simulink model "my_queue_system"  (R2023a)
settings: Solver=VariableStepAuto  StartTime=0.0  StopTime=1000  RelTol=1e-3
values from neighbouring files (symbols this model uses):
  m = m + 1    (= 2)    [TMO5liubimov.m]    (also in laba2.m = 14; laba3.m = 200; test.m = 5)
  n = 31    [laba2.m]    (also in test.m = 7)
settings Model: PacingRate=14  Creator=PC  LastModifiedBy=PC

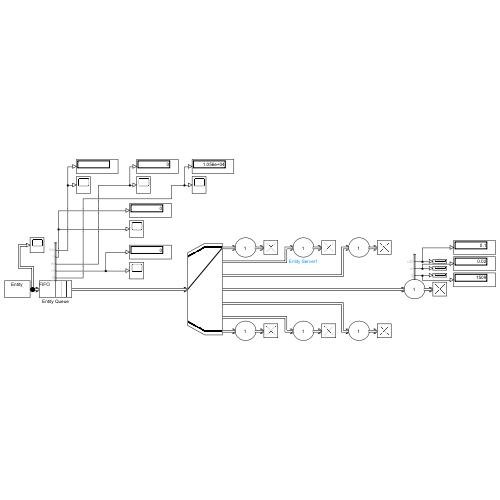
[thumbnail: Simulink's stored preview of the top-level diagram]
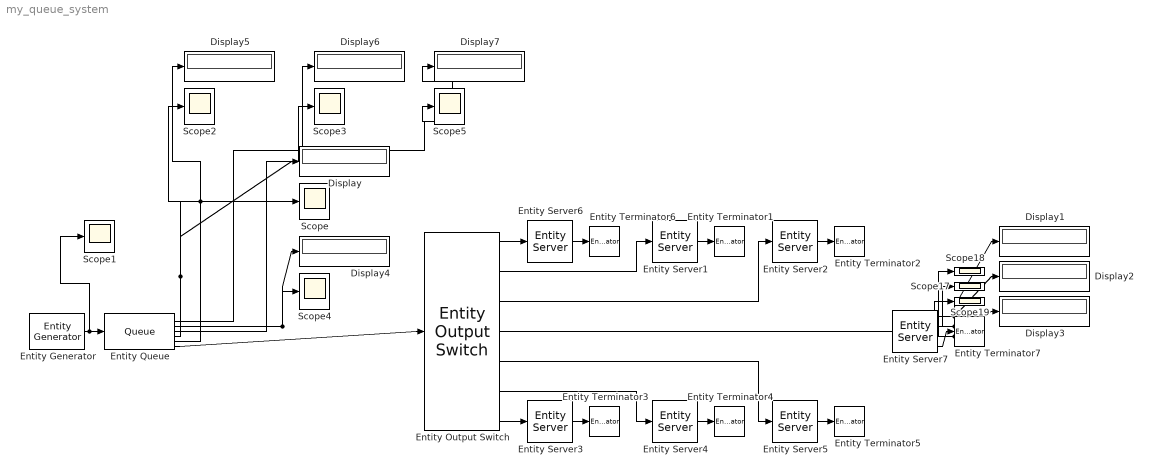
== system my_queue_system ==
  Display{,1..7} (8 alike) : Display
  Entity Output Switch : EntityOutputSwitch  InputPortMessageModes=m  OutputPortMessageModes=m,m,m,m,m,m,m  NumberOutputPorts=7  SwitchingCriterion=Round robin  SwitchAttributeName=Attribute1
      settings: OutputPortMap=o0,o1,o2,o3,o4,o5,o6
  Entity Generator : EntityGenerator  OutputPortMessageModes=m  Period=1/35  GenerateEntityAtSimulationStart=off  EntityType=Structured  EntityTypeName=Entity
  Entity Queue : Queue  InputPortMessageModes=m  OutputPortMessageModes=n,n,n,n,n,m  Capacity=5  NumberEntitiesDeparted=on  NumEntitiesExtracted=on  NumberEntitiesInBlock=on  AverageWait=on  AverageQueueLength=on
      settings: OutputPortMap=o0,o1,o2,o3,o7,o5
  Entity Server{1..6} (6 alike) : EntityServer  InputPortMessageModes=m  OutputPortMessageModes=m  Capacity=1  ServiceTimeValue=1/50
  Entity Server7 : EntityServer  InputPortMessageModes=m  OutputPortMessageModes=n,n,n,m  Capacity=1  ServiceTimeValue=1/50  NumberEntitiesDeparted=on  AverageWait=on  Utilization=on
      settings: OutputPortMap=o0,o4,o5,o9
  Entity Terminator{1..7} (7 alike) : EntityTerminator  InputPortMessageModes=m
  Scope{,1..5,17..19} (9 alike) : Scope
  wires:
  Entity Server6/1 -> Entity Terminator6/1
  Entity Server1/1 -> Entity Terminator1/1
  Entity Server2/1 -> Entity Terminator2/1
  Entity Server3/1 -> Entity Terminator3/1
  Entity Server4/1 -> Entity Terminator4/1
  Entity Server5/1 -> Entity Terminator5/1
  Entity Server7/4 -> Entity Terminator7/1
  Entity Server7/2 -> Display2/1, Scope17/1
  Entity Server7/3 -> Display1/1, Scope18/1
  Entity Server7/1 -> Scope19/1, Display3/1
  Entity Generator/1 -> Scope1/1, Entity Queue/1
  Entity Output Switch/4 -> Entity Server7/1
  Entity Output Switch/7 -> Entity Server3/1
  Entity Output Switch/1 -> Entity Server6/1
  Entity Output Switch/2 -> Entity Server1/1
  Entity Output Switch/3 -> Entity Server2/1
  Entity Output Switch/6 -> Entity Server4/1
  Entity Output Switch/5 -> Entity Server5/1
  Entity Queue/2 -> Display4/1, Scope4/1
  Entity Queue/4 -> Display/1, Scope/1
  Entity Queue/6 -> Entity Output Switch/1
  Entity Queue/5 -> Display5/1, Scope2/1
  Entity Queue/3 -> Display6/1, Scope3/1
  Entity Queue/1 -> Display7/1, Scope5/1
